simulink model "group7"  (R2022b)
settings: Solver=FixedStepAuto  StartTime=0.0  StopTime=100.0  RelTol=1e-3
libraries: robotlib x8
settings Model: Creator=katiegildersleeve  LastModifiedBy=sprinkle
settings OptimizationCC: EnhancedBackFolding=on  PassReuseOutputArgsAs=Individual arguments  ZeroExternalMemoryAtStartup=off  ZeroInternalMemoryAtStartup=off  MaxStackSize=64  OptimizeBlockOrder=speed  DifferentSizesBufferReuse=on  OptimizationCustomize=off  EfficientTunableParamExpr=on
settings DebuggingCC: ParameterTunabilityLossMsg=error
settings HardwareCC: ProdBitPerPointer=32  ProdBitPerSizeT=32  ProdBitPerPtrDiffT=32  ProdLargestAtomicFloat=None  ProdIntDivRoundTo=Undefined  ProdEndianess=Unspecified  ProdWordSize=32  ProdHWDeviceType=Generic->Unspecified (assume 32-bit Generic)  UseEmbeddedCoderFeatures=off
settings SFSimCC: MATLABDynamicMemAlloc=off
settings RTWCC: Description=Embedded Coder  SystemTargetFile=ert.tlc  HardwareBoard=Robot Operating System (ROS)  TLCOptions="-aInlineSetEventsForThisBaseRateFcn=TLC_FALSE -aSuppressMultiTaskScheduler=TLC_FALSE  -aRateBasedStepFcn=0"  TemplateMakefile=ert_default_tmf  Toolchain=Catkin  TargetLang=C++  GPUComputeCapability=5.0
settings CodeAppCC: ForceParamTrailComments=on  IgnoreCustomStorageClasses=off  OperatorAnnotations=on  SimulinkDataObjDesc=on  SFDataObjDesc=on  InsertBlockDesc=on
settings ERTTargetCC: SupportNonInlinedSFcns=on

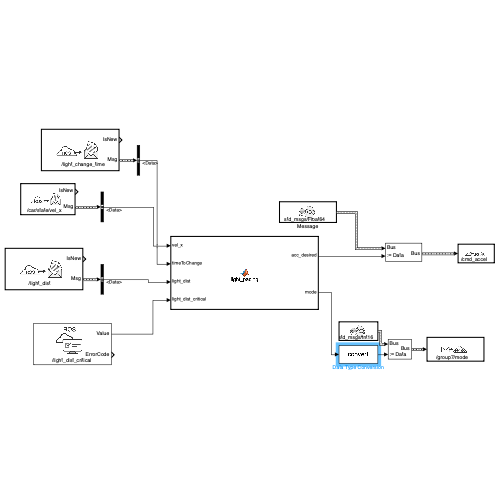
[thumbnail: Simulink's stored preview of the top-level diagram]
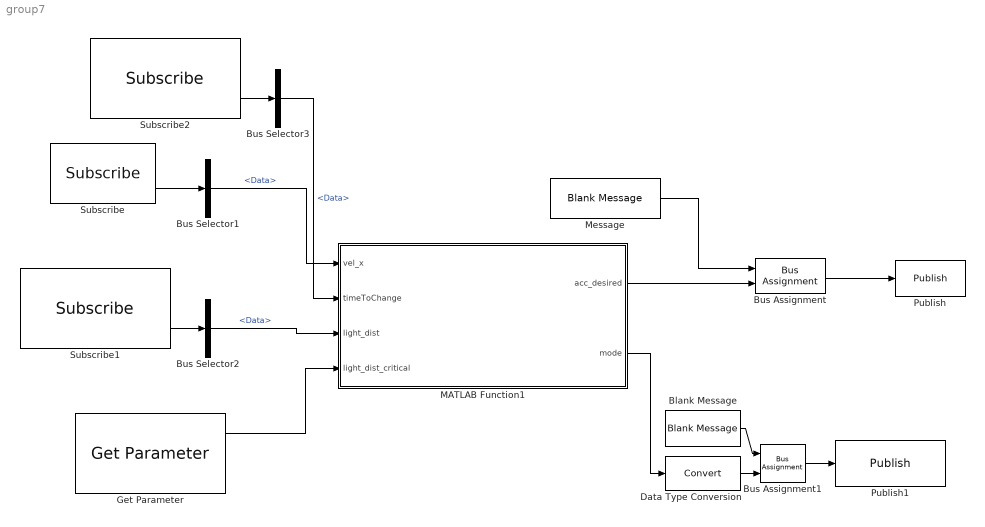
== system group7 ==
  Blank Message : robotlib/Blank Message  messageClass=Message  entityType=std_msgs/Int16  messageType=std_msgs/Int16  SampleTime=inf  legacyBusStruct=off
      settings: LibrarySourceBlock=roslib/ROS/Blank Message
  Bus Assignment : BusAssignment  AssignedSignals=Data
  Bus Assignment1 : BusAssignment  AssignedSignals=Data
  Bus Selector1 : BusSelector  OutputSignals=Data
  Bus Selector2 : BusSelector  OutputSignals=Data
  Bus Selector3 : BusSelector  OutputSignals=Data
  Data Type Conversion : DataTypeConversion  SaturateOnIntegerOverflow=off  RndMeth=Floor
  Get Parameter : robotlib/Get Parameter  ParameterSource=Specify your own  ParameterName=/light_dist_critical  ParameterType=double  ParameterMaxArrayLength=16  ParameterInitialValue=100.0  SampleTime=-1  ShowErrorCodeOutput=on  ModelName=group7  BlockId=ParamGet_group7_68
      settings: LibrarySourceBlock=roslib/ROS/Get Parameter
  MATLAB Function1 : MATLAB Function  TreatAsAtomicUnit=on
  Message : robotlib/Blank Message  messageClass=Message  entityType=std_msgs/Float64  messageType=std_msgs/Float64  SampleTime=inf  legacyBusStruct=off
  Publish : robotlib/Publish  topicSource=Specify your own  topic=/cmd_accel  messageType=std_msgs/Float64  legacyBusStruct=off  messageQueueLength=1
  Publish1 : robotlib/Publish  topicSource=Specify your own  topic=/group7/mode  messageType=std_msgs/Int16  legacyBusStruct=off  messageQueueLength=1
      settings: LibrarySourceBlock=roslib/ROS/Publish
  Subscribe : robotlib/Subscribe  topicSource=Specify your own  topic=/car/state/vel_x  messageType=std_msgs/Float64  SampleTime=-1  legacyBusStruct=off  messageQueueLength=1
  Subscribe1 : robotlib/Subscribe  topicSource=Specify your own  topic=/light_dist  messageType=std_msgs/Float64  SampleTime=-1  legacyBusStruct=off  messageQueueLength=1
      settings: LibrarySourceBlock=roslib/ROS/Subscribe
  Subscribe2 : robotlib/Subscribe  topicSource=Specify your own  topic=/light_change_time  messageType=std_msgs/Float64  SampleTime=-1  legacyBusStruct=off  messageQueueLength=1
      settings: LibrarySourceBlock=roslib/ROS/Subscribe
  wires:
  Message/1 -> Bus Assignment/1
  Bus Assignment/1 -> Publish/1
  MATLAB Function1/1(acc_desired) -> Bus Assignment/2
  MATLAB Function1/2(mode) -> Data Type Conversion/1
  Bus Selector2/1 -> MATLAB Function1/3(light_dist)  "<Data>"
  Subscribe/2 -> Bus Selector1/1
  Bus Selector1/1 -> MATLAB Function1/1(vel_x)  "<Data>"
  Get Parameter/1 -> MATLAB Function1/4(light_dist_critical)
  Subscribe1/2 -> Bus Selector2/1
  Subscribe2/2 -> Bus Selector3/1
  Bus Selector3/1 -> MATLAB Function1/2(timeToChange)  "<Data>"
  Blank Message/1 -> Bus Assignment1/1
  Bus Assignment1/1 -> Publish1/1
  Data Type Conversion/1 -> Bus Assignment1/2

== matlab function group7/MATLAB Function1 ==
  data: vel_x input; timeToChange input; acc_desired output; mode output; light_dist input; light_dist_critical input
function [acc_desired, mode] = light_pacing(vel_x, timeToChange, light_dist, light_dist_critical)

    % JMS: this is calculated better in the model
    % Read the current simulation time and stop light distance from input
    %time_step = 1;
    %sim_time = sim_time_read;

    % using old var names but more consistent input names
    stop_light_distance = light_dist;
    vel_ego = vel_x;

    % JMS: this is calculated better in the model
    % Traffic Light Timing
    %
    % time_to_green = 40 - sim_time;  % Time until the light turns green
    time_to_green = timeToChange;

    % Control Parameters
    alpha = 0.25;         % Control gain

    % JMS: this is calculated better in the model
    % Update the distance to the stoplight based on velocity
    %stop_light_distance = stop_light_distance - (vel_ego * time_step);

    % Check for critical distance to the lead vehicle (space_gap) or stoplight
    critical_distance_to_stoplight = light_dist_critical;    % Distance to start slowing down for the stoplight

    mode=0;
    % If the light is too close, slow down to be able to time better
    if stop_light_distance <= critical_distance_to_stoplight && time_to_green > 0
        % Approaching the stoplight while it's red
        % Calculate target velocity to arrive as the light turns green
        target_velocity = stop_light_distance / time_to_green;
        acc_desired = alpha * (target_velocity - vel_ego);
        mode=1;
    else
        % continue on as if nothing happened
        mode=0;
        % Normal control behavior (no immediate lead vehicle or red light)
        acc_desired = alpha * (15 - vel_ego);
    end

    % Safety Check: Prevent negative or excessively high acceleration
    if stop_light_distance < 0
        mode=2;
        acc_desired = alpha * (15 - vel_ego);  % Stop if too close to the stoplight
    end

    % JMS: this is calculated better in the model
    % Update the simulation time
    %sim_time = sim_time + time_step;

    % JMS: this is calculated better in the model
    % Output the updated values
    %sim_time_out = sim_time;
    %stop_light_distance_out = stop_light_distance;
end
